simulink model "SMC"  (R2025b)
settings: Solver=VariableStepAuto  StartTime=0.0  StopTime=10.0  RelTol=1e-3
InitFcn:
  | run("init.m");
values from neighbouring files (symbols this model uses):
  B = [-1 0 -1; 1 0 0; 0 1 -1; 0 0 1]    [init.m]
  dq_init = [0;0;0;0]    [init.m]
  q_init = [pi/2 + 0.05; 0; K.q2_ref; 0]    [init.m]
settings Model: Creator=Acer  LastModifiedBy=Acer

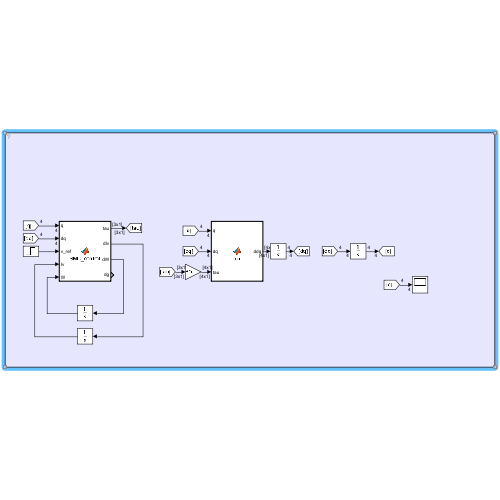
[thumbnail: Simulink's stored preview of the top-level diagram]
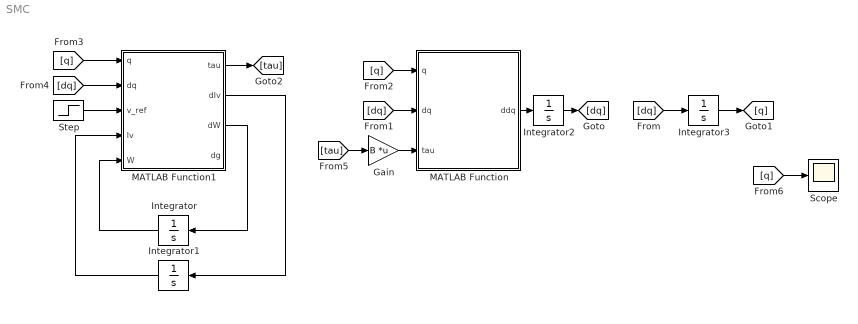
== system SMC ==
  Gain : Gain  Gain=B  Multiplication=Matrix(K*u)
  Integrator : Integrator
  Integrator1 : Integrator
  Integrator2 : Integrator  InitialCondition=dq_init
  Integrator3 : Integrator  InitialCondition=q_init
  MATLAB Function : MATLAB Function  TreatAsAtomicUnit=on
  MATLAB Function1 : MATLAB Function  TreatAsAtomicUnit=on
  Scope : Scope
      settings: ActiveDisplayYMinimum=-5.7207347307707908  ActiveDisplayYMaximum=48.486612241213045
  Step : Step  After=0.6  SampleTime=0
  wires:
  MATLAB Function1/3(dW) -> Integrator/1
  Integrator/1 -> MATLAB Function1/5(W)
  MATLAB Function1/2(dIv) -> Integrator1/1
  Integrator1/1 -> MATLAB Function1/4(Iv)
  MATLAB Function/1(ddq) -> Integrator2/1
  Integrator2/1 -> [dq]
  [dq] -> Integrator3/1
  Integrator3/1 -> [q]
  [q] -> MATLAB Function/1(q)
  [dq] -> MATLAB Function/2(dq)
  MATLAB Function1/1(tau) -> [tau]
  [q] -> MATLAB Function1/1(q)
  [dq] -> MATLAB Function1/2(dq)
  Step/1 -> MATLAB Function1/3(v_ref)
  [q] -> Scope/1
  [tau] -> Gain/1
  Gain/1 -> MATLAB Function/3(tau)

== matlab function SMC/MATLAB Function1 ==
  data: q input; tau output; dq input; v_ref input; dIv output; dW output; dg output; Iv input; W input; K parameter
function [tau, dIv, dW, dg] = SMC_control(q,      dq,      v_ref, Iv, W, K)


[tau, dIv, dW, dg] = wbr_ctrl(q,  dq, v_ref, Iv, W, K);

== matlab function SMC/MATLAB Function ==
  data: q input; ddq output; dq input; tau input; B parameter
function ddq = fcn(q,dq, tau, B)

[M,CdQ, Gv] = calc_dynamics(q,dq);

ddq = M\(-CdQ - Gv + tau);
